simulink model "Final_Project_Control"  (R2023b)
settings: Solver=VariableStepAuto  StartTime=0.0  StopTime=0.5  RelTol=1e-6
values from neighbouring files (symbols this model uses):
  C = 22e-6    (= 2.2e-05)    [Final_Project.m]
  fs = 12e3    (= 12000)    [Final_Project.m]
  Gc_Den = cell2mat(Gc.Denominator)    [Final_Project.m]
  Gc_Num = cell2mat(Gc.Numerator)    [Final_Project.m]
  L = 1e-3    (= 0.001)    [Final_Project.m]
  R = 22    [Final_Project.m]
  Tds_Den = cell2mat(Tds.Denominator)    [Final_Project.m]
  Tds_Num = cell2mat(Tds.Numerator)    [Final_Project.m]
  Vd = 36*sqrt(2)    [Final_Project.m]
libraries: spsSeriesRLCBranchLib x3, spsVoltageMeasurementLib x2, spsCurrentMeasurementLib x1, spsDiodeLib x1, spsIdealSwitchLib x1, spsMeanLib x1, eePwmGenerator x1, spsControlledVoltageSourceLib x1, spspowerguiLib x1
settings Model: Creator=lucas  LastModifiedBy=Lucas
settings SolverCC: ZeroCrossAlgorithm=Adaptive
settings DebuggingCC: AlgebraicLoopMsg=none  IgnoredZcDiagnostic=none

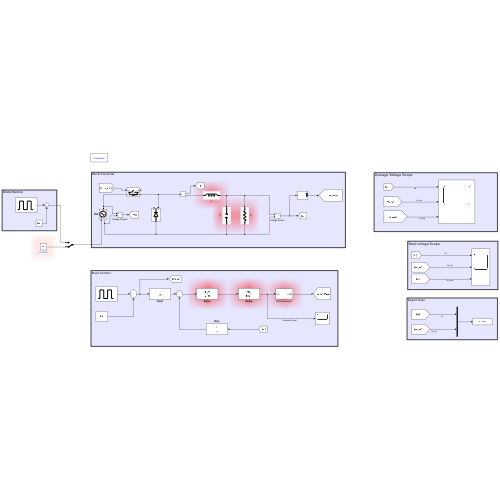
[thumbnail: Simulink's stored preview of the top-level diagram]
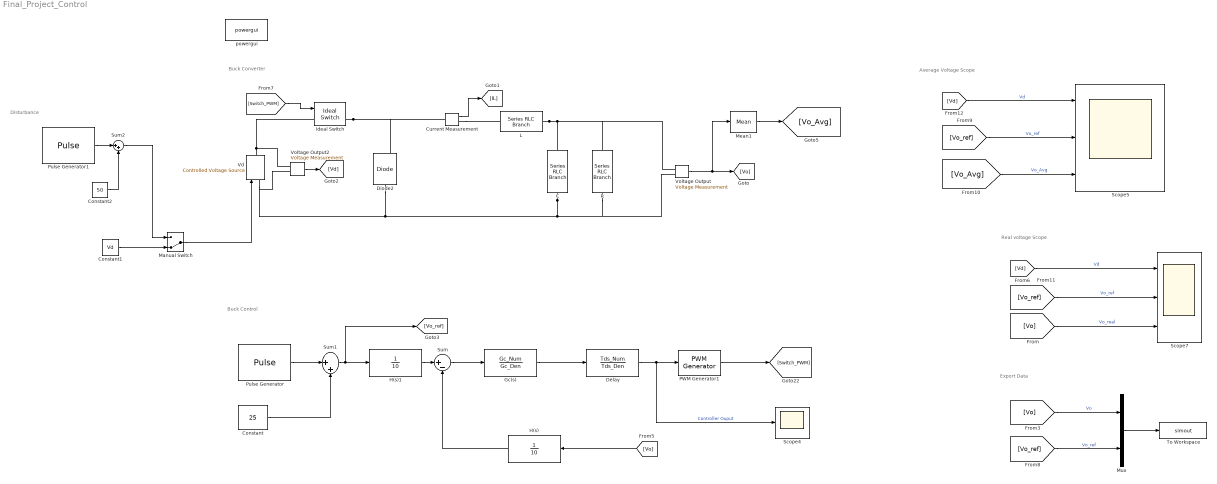
== system Final_Project_Control ==
  note: Export Data
  note: Disturbance
  note: Real voltage Scope
  note: Average Voltage Scope
  note: Buck Control
  note: Buck Converter
  C : spsSeriesRLCBranchLib/Series RLC Branch  LConnTagsString=__new0  RConnTagsString=__new0  BranchType=C  Resistance=1  Inductance=L  SetiL0=off  InitialCurrent=0  Capacitance=C  Setx0=off  InitialVoltage=0  Measurements=None
  Constant : Constant  Value=25
  Constant1 : Constant  Value=Vd
  Constant2 : Constant  Value=50
  Current Measurement : spsCurrentMeasurementLib/Current Measurement  PhasorSimulation=off  OutputType=Complex  PSBequivalent=0
  Delay : TransferFcn  Numerator=Tds_Num  Denominator=Tds_Den
  Diode2 : spsDiodeLib/Diode  Ron=0.00001  Lon=0  Vf=0  IC=0  UseSnubber=0  Rs=inf  Cs=inf  Measurements=on
  Gc(s) : TransferFcn  Numerator=Gc_Num  Denominator=Gc_Den
  H(s) : TransferFcn  Denominator=[10]
  H(s)1 : TransferFcn  Denominator=[10]
  Ideal Switch : spsIdealSwitchLib/Ideal Switch  Ron=0.001  Lon=0  IC=0  Rs=1e5  Cs=inf  Measurements=on
  L : spsSeriesRLCBranchLib/Series RLC Branch  LConnTagsString=__new0  RConnTagsString=__new0  BranchType=L  Resistance=1  Inductance=L  SetiL0=off  InitialCurrent=0  Capacitance=1e-6  Setx0=off  InitialVoltage=0  Measurements=None
  Manual Switch : ManualSwitch  CurrentSetting=0
  Mean1 : spsMeanLib/Mean  Freq=60  Vinit=0  Ts=0
  Mux : Mux  Inputs=2
  PWM Generator1 : eePwmGenerator/PWM Generator  CarrCount=Up  Tper=1/fs  Tdelay=0.5/fs  Ts=0
  Pulse Generator : DiscretePulseGenerator  PulseType=Time based  Amplitude=20  Period=0.5  PulseWidth=50  PhaseDelay=0.2
  Pulse Generator1 : DiscretePulseGenerator  PulseType=Time based  Amplitude=20  Period=0.5  PulseWidth=50  PhaseDelay=0.1
  R : spsSeriesRLCBranchLib/Series RLC Branch  LConnTagsString=__new0  RConnTagsString=__new0  BranchType=R  Resistance=R  Inductance=L  SetiL0=off  InitialCurrent=0  Capacitance=1e-6  Setx0=off  InitialVoltage=0  Measurements=None
  Scope4 : Scope
  Scope5 : Scope  NumInputPorts=3
  Scope7 : Scope  NumInputPorts=3
  Sum : Sum  Inputs=|+-
  Sum1 : Sum  Inputs=|++
  Sum2 : Sum  Inputs=|++
  To Workspace : ToWorkspace  VariableName=simout  SaveFormat=Structure With Time  SampleTime=-1
  Vd : spsControlledVoltageSourceLib/Controlled Voltage Source  Initialize=on  Source_Type=DC  Amplitude=50  Phase=0  Frequency=0  Measurements=None
  Voltage Output : spsVoltageMeasurementLib/Voltage Measurement  PhasorSimulation=off  OutputType=Complex  PSBequivalent=0
  Voltage Output2 : spsVoltageMeasurementLib/Voltage Measurement  PhasorSimulation=off  OutputType=Complex  PSBequivalent=0
  powergui : spspowerguiLib/powergui  Priority=1  SimulationMode=Continuous  SampleTime=50e-6  frequency=60  Iterations=50  frequencyindice=0  Pbase=100e6  ErrMax=1e-4  UnitsV=kV  UnitsW=MW  buscounter=0  FunctionMessages=off  echomessages=off  EnableUseOfTLC=off  CurrentSourceSwitches=off  DisableSnubberDevices=off  DisableRonSwitches=off  DisableVfSwitches=off  DisplayEquations=off  AutomaticDiscreteSolvers=off  SolverType=Tustin/Backward Euler (TBE)  Interpol=off  ExternalGateDelay=off  methode=off  Ts=100  x0status=blocks  SPID=on  SwTol=0  HookPort=off  NonlinearTolerance=1e-4  nMaxIteration=100  ContinueOnMaxIteration=off  RestoreLinks=warning  ResistiveCurrentMeasurement=off  Frange=[0:2:500]  Ylog=off  Xlog=on  ShowGrid=off  save=off  variable=ZData  structure=0  ZoomFFT=off  StartTime=0.0  cycles=1  DisplayStyle=1  fundamental=60  FreqAxis=off  MaxFrequency=1000  frequencyindicesteady=1  RmsSteady=1  display=off
  wires:
  [Switch_PWM] -> Ideal Switch/1
  Sum/1 -> Gc(s)/1
  Current Measurement/1 -> [IL]
  Sum1/1 -> [Vo_ref], H(s)1/1
  Voltage Output/1 -> Mean1/1, [Vo]
  Constant/1 -> Sum1/2
  Pulse Generator/1 -> Sum1/1
  Mean1/1 -> [Vo_Avg]
  [Vo_ref] -> Scope7/2  "Vo_ref"
  [Vo] -> Scope7/3  "Vo_real"
  Voltage Output2/1 -> [Vd]
  Pulse Generator1/1 -> Sum2/1
  Manual Switch/1 -> Vd/1
  Constant1/1 -> Manual Switch/2
  Sum2/1 -> Manual Switch/1
  Constant2/1 -> Sum2/2
  [Vo_ref] -> Scope5/2  "Vo_ref"
  [Vo_Avg] -> Scope5/3  "Vo_Avg"
  [Vd] -> Scope5/1  "Vd"
  [Vo] -> H(s)/1
  H(s)/1 -> Sum/2
  Gc(s)/1 -> Delay/1
  Delay/1 -> Scope4/1, PWM Generator1/1  "Controller Ouput"
  PWM Generator1/1 -> [Switch_PWM]
  H(s)1/1 -> Sum/1
  [Vd] -> Scope7/1  "Vd"
  [Vo] -> Mux/1  "Vo"
  [Vo_ref] -> Mux/2  "Vo_ref"
  Mux/1 -> To Workspace/1
  connections:
  Ideal Switch/RConn1 -- Current Measurement/LConn1 -- Diode2/RConn1
  C/RConn1 -- Voltage Output/LConn2 -- R/RConn1 -- Voltage Output2/LConn2 -- Vd/LConn1 -- Diode2/LConn1
  L/RConn1 -- Voltage Output/LConn1 -- R/LConn1 -- C/LConn1
  Current Measurement/RConn1 -- L/LConn1
  Vd/RConn1 -- Ideal Switch/LConn1 -- Voltage Output2/LConn1
